simulink model "FINAL_MODEL"  (R2021b)
settings: Solver=VariableStepAuto  StartTime=0.0  StopTime=200  RelTol=1e-3
values from neighbouring files (symbols this model uses):
  lr = 1.6    [projectsetup.m]
  m = 1521    [projectsetup.m]
  posSelector = [1,0,0,0,0,0; 0,0,1,0,0,0]    [projectsetup.m]
  tau = 0.5    [projectsetup.m]
  Ts = 0.1    [projectsetup.m]
  x0_ego = 0    [projectsetup.m]
undefined symbols (not defined in the file or in its folder): AEB, driving
libraries: drivingscenarioandsensors x3, slpidlib x1, trackingutilitieslib x1, drivinglib x1, autolibshared x1
settings Model: Creator=DELL  LastModifiedBy=gioge

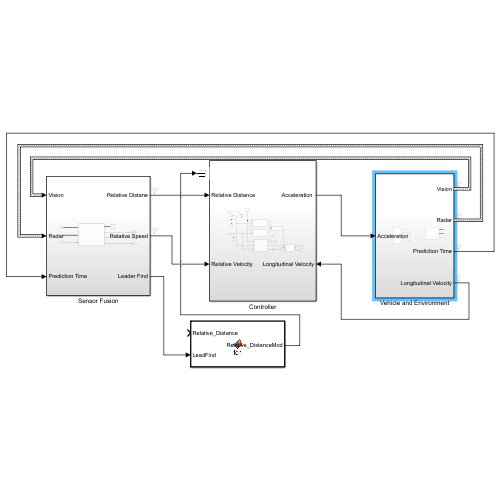
[thumbnail: Simulink's stored preview of the top-level diagram]
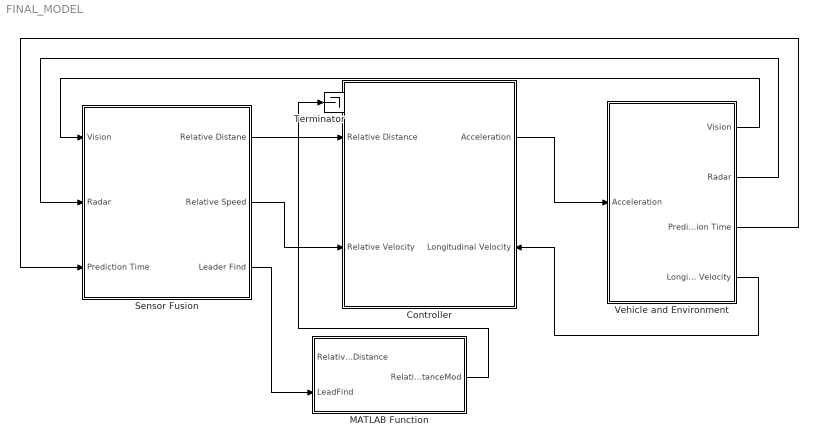
== system FINAL_MODEL ==
  Controller : Subsystem
      settings: PortSchema="{\"entries\":[{\"content\":{\"sides\":[{\"content\":{\"connectorIds\":[\"In1\",\"In2\"]},\"type\":\"ConnectorPlacement.EquallySpacedRectSide\",\"uuid\":\"09646beb-0eff-4bcf-8a55-80fd4dda4f7a\"},{\"content\":{\"connectorIds\":[\"Out1\",\"In3\"],\"side\":\"RIGHT\"},\"type\":\"ConnectorPlacement.EquallySpacedRectSide\",\"uuid\":\"ec392ed6-633f-4d34-b95c-b5fe46f60e49\"},{\"content\":{\"connectorIds\":[],\"side\":\"TOP\"},\"type\":\"ConnectorPlacement.EquallySpacedRectSide\",\"uuid\":\"4c514b4e-b507-45d4-96c7-33bdb79faf54\"},{\"content\":{\"connectorIds\":[],\"side\":\"BOTTOM\"},\"type\":\"ConnectorPlacement.EquallySpacedRectSide\",\"uuid\":\"07bcd855-5437-489d-a027-c45770d5736d\"}]},\"type\":\"ConnectorPlacement.EquallySpacedConnector\",\"uuid\":\"1e09dc8d-e6d5-4259-816a-8e498a37a0b4\"}],\"packageUris\":[\"http://schema.mathworks.com/mf0/Connector/R2020b\"],\"version\":\"1.0\"}"
  MATLAB Function : MATLAB Function  TreatAsAtomicUnit=on
  Sensor Fusion : Subsystem
  Terminator : Terminator
  Vehicle and Environment : Subsystem
  wires:
  Vehicle and Environment/3(Prediction Time) -> Sensor Fusion/3(Prediction Time)
  Vehicle and Environment/2(Radar) -> Sensor Fusion/2(Radar)
  Vehicle and Environment/1(Vision) -> Sensor Fusion/1(Vision)
  Vehicle and Environment/4(Longitudinal Velocity) -> Controller/3(Longitudinal Velocity)
  Sensor Fusion/1(Relative Distane) -> Controller/1(Relative Distance)
  Sensor Fusion/2(Relative Speed) -> Controller/2(Relative Velocity)
  Controller/1("Acceleration ") -> Vehicle and Environment/1(Acceleration)
  Sensor Fusion/3(Leader Find) -> MATLAB Function/2(LeadFind)
  MATLAB Function/1(Relative_DistanceMod) -> Terminator/1

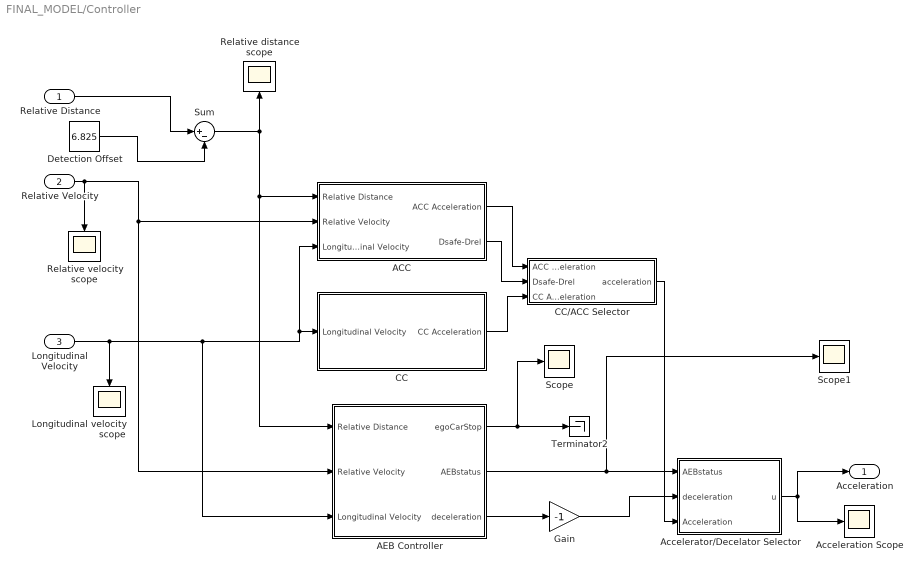
== system FINAL_MODEL/Controller ==
  Relative Distance : Inport
  Relative Velocity : Inport  Port=2
  Longitudinal Velocity : Inport  Port=3
  ACC : Subsystem
  AEB Controller : Subsystem
  Acceleration Scope : Scope
  Accelerator/Decelator Selector : Subsystem
  CC : Subsystem
  CC/ACC Selector : Subsystem
  Detection Offset : Constant  Value=6.825
  Gain : Gain  Gain=-1
  Longitudinal velocity scope : Scope
  Relative distance scope : Scope
  Relative velocity scope : Scope
  Scope : Scope
  Scope1 : Scope
  Sum : Sum  Inputs=|+-
  Terminator2 : Terminator
  "Acceleration " : Outport  OutDataTypeStr=double  PortDimensions=1  SampleTime=[0.10000000000000001,0]  VectorParamsAs1DForOutWhenUnconnected=off
  wires:
  Relative Velocity/1 -> Relative velocity scope/1, AEB Controller/2(Relative Velocity), ACC/2(Relative Velocity)
  Relative Distance/1 -> Sum/1
  AEB Controller/1(egoCarStop) -> Scope/1, Terminator2/1
  AEB Controller/2(AEBstatus) -> Scope1/1, Accelerator/Decelator Selector/1(AEBstatus)
  AEB Controller/3(deceleration) -> Gain/1
  Longitudinal Velocity/1 -> AEB Controller/3(Longitudinal Velocity), ACC/3(Longitudinal Velocity), CC/1(Longitudinal Velocity), Longitudinal velocity scope/1
  Sum/1 -> AEB Controller/1(Relative Distance), ACC/1(Relative Distance), Relative distance scope/1
  Detection Offset/1 -> Sum/2
  Accelerator/Decelator Selector/1(u) -> "Acceleration "/1, Acceleration Scope/1
  Gain/1 -> Accelerator/Decelator Selector/2(deceleration)
  ACC/1(ACC Acceleration) -> CC/ACC Selector/1(ACC Acceleration)
  ACC/2(Dsafe-Drel) -> CC/ACC Selector/2(Dsafe-Drel)
  CC/1(CC Acceleration) -> CC/ACC Selector/3(CC Acceleration)
  CC/ACC Selector/1(acceleration) -> Accelerator/Decelator Selector/3(Acceleration)

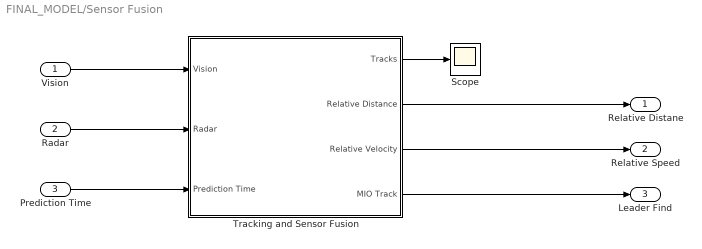
== system FINAL_MODEL/Sensor Fusion ==
  Vision : Inport  OutDataTypeStr=Bus: BusVision  PortDimensions=[1 1]  SampleTime=[0.10000000000000001,0]  BusOutputAsStruct=on
  Radar : Inport  Port=2  OutDataTypeStr=Bus: BusRadar  PortDimensions=[1 1]  SampleTime=[0.10000000000000001,0]  BusOutputAsStruct=on
  Prediction Time : Inport  Port=3  OutDataTypeStr=double  PortDimensions=[1 1]  SampleTime=[0.10000000000000001,0]  BusOutputAsStruct=on
  Scope : Scope
  Tracking and Sensor Fusion : Subsystem  TreatAsAtomicUnit=on
      settings: RTWFileNameOpts=Use function name
  Relative Distane : Outport  OutDataTypeStr=double  PortDimensions=1  SampleTime=[0.10000000000000001,0]  VectorParamsAs1DForOutWhenUnconnected=off  BusOutputAsStruct=on
  Relative Speed : Outport  Port=2  OutDataTypeStr=double  PortDimensions=1  SampleTime=[0.10000000000000001,0]  VectorParamsAs1DForOutWhenUnconnected=off  BusOutputAsStruct=on
  Leader Find : Outport  Port=3  OutDataTypeStr=double  PortDimensions=1  SampleTime=[0.10000000000000001,0]  VectorParamsAs1DForOutWhenUnconnected=off  BusOutputAsStruct=on
  wires:
  Tracking and Sensor Fusion/2(Relative Distance) -> Relative Distane/1
  Prediction Time/1 -> Tracking and Sensor Fusion/3(Prediction Time)
  Tracking and Sensor Fusion/3(Relative Velocity) -> Relative Speed/1
  Tracking and Sensor Fusion/1(Tracks) -> Scope/1
  Radar/1 -> Tracking and Sensor Fusion/2(Radar)
  Vision/1 -> Tracking and Sensor Fusion/1(Vision)
  Tracking and Sensor Fusion/4(MIO Track) -> Leader Find/1

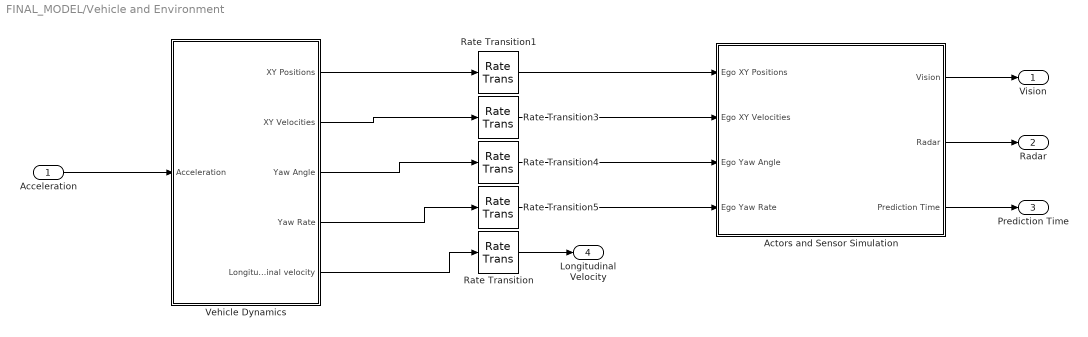
== system FINAL_MODEL/Vehicle and Environment ==
  Acceleration : Inport
  Actors and Sensor Simulation : Subsystem
  Rate Transition{,1,3..5} (5 alike) : RateTransition  OutPortSampleTime=Ts
  Vehicle Dynamics : Subsystem  VariantControl=Variant2
  Vision : Outport  VectorParamsAs1DForOutWhenUnconnected=off
  Radar : Outport  Port=2  VectorParamsAs1DForOutWhenUnconnected=off
  Prediction Time : Outport  Port=3  VectorParamsAs1DForOutWhenUnconnected=off
  Longitudinal Velocity : Outport  Port=4  VectorParamsAs1DForOutWhenUnconnected=off
  wires:
  Acceleration/1 -> Vehicle Dynamics/1(Acceleration)
  Vehicle Dynamics/5(Longitudinal velocity) -> Rate Transition/1
  Vehicle Dynamics/1(XY Positions) -> Rate Transition1/1
  Vehicle Dynamics/3(Yaw Angle) -> Rate Transition4/1
  Actors and Sensor Simulation/1(Vision) -> Vision/1
  Rate Transition/1 -> Longitudinal Velocity/1
  Vehicle Dynamics/2(XY Velocities) -> Rate Transition3/1
  Rate Transition4/1 -> Actors and Sensor Simulation/3(Ego Yaw Angle)
  Actors and Sensor Simulation/2(Radar) -> Radar/1
  Rate Transition1/1 -> Actors and Sensor Simulation/1(Ego XY Positions)
  Rate Transition5/1 -> Actors and Sensor Simulation/4(Ego Yaw Rate)
  Rate Transition3/1 -> Actors and Sensor Simulation/2(Ego XY Velocities)
  Actors and Sensor Simulation/3(Prediction Time) -> Prediction Time/1
  Vehicle Dynamics/4(Yaw Rate) -> Rate Transition5/1

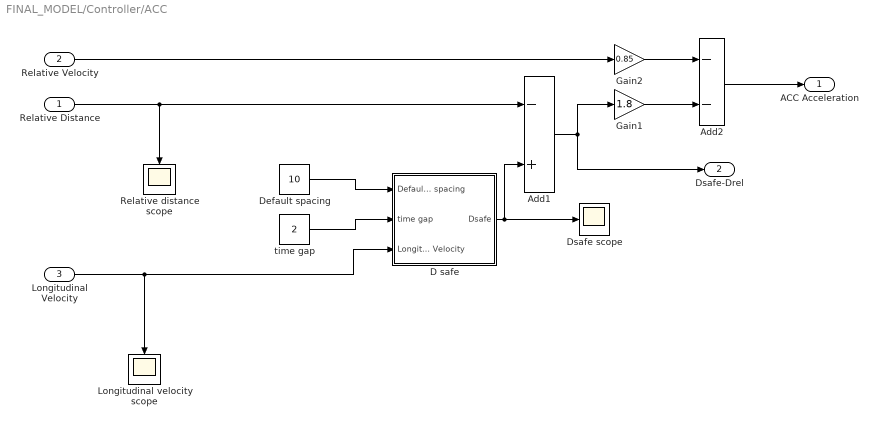
== system FINAL_MODEL/Controller/ACC ==
  Relative Distance : Inport
  Relative Velocity : Inport  Port=2
  Longitudinal Velocity : Inport  Port=3
  Add1 : Sum  Inputs=-+
  Add2 : Sum  Inputs=--
  D safe : Subsystem
  Default spacing : Constant  Value=10
  Dsafe scope : Scope
  Gain1 : Gain  Gain=1.8
  Gain2 : Gain  Gain=0.85
  Longitudinal velocity scope : Scope
  Relative distance scope : Scope
  time gap : Constant  Value=2
  ACC Acceleration : Outport
  Dsafe-Drel : Outport  Port=2
  wires:
  Add1/1 -> Dsafe-Drel/1, Gain1/1
  Relative Distance/1 -> Add1/1, Relative distance scope/1
  D safe/1(Dsafe) -> Add1/2, Dsafe scope/1
  Relative Velocity/1 -> Gain2/1
  time gap/1 -> D safe/2(time gap)
  Longitudinal Velocity/1 -> Longitudinal velocity scope/1, D safe/3(Longitudinal Velocity)
  Default spacing/1 -> D safe/1(Default spacing)
  Gain2/1 -> Add2/1
  Gain1/1 -> Add2/2
  Add2/1 -> ACC Acceleration/1

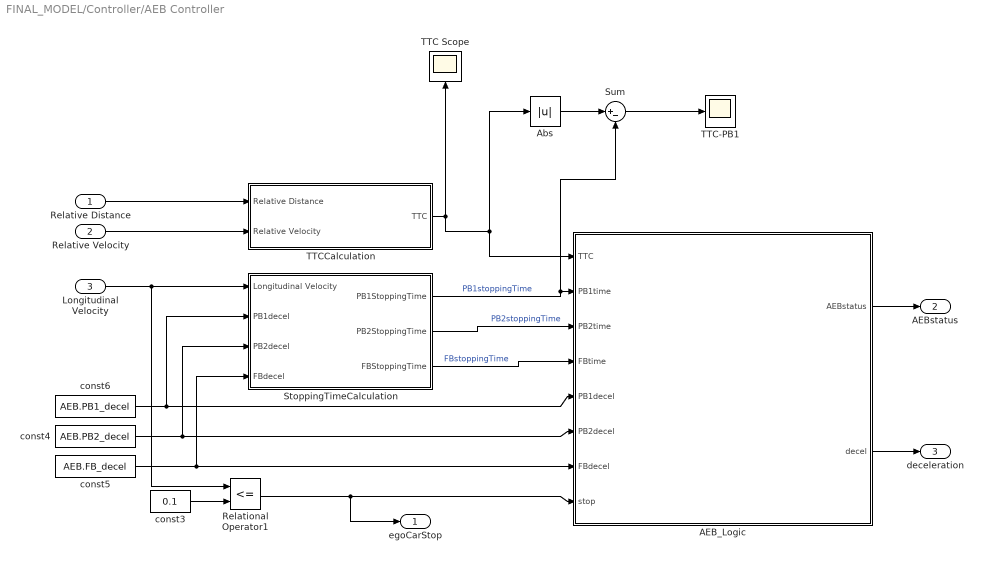
== system FINAL_MODEL/Controller/AEB Controller ==
  Relative Distance : Inport
  Relative Velocity : Inport  Port=2
  Longitudinal Velocity : Inport  Port=3
  AEB_Logic : Stateflow chart  TreatAsAtomicUnit=on
  Abs : Abs
  Relational Operator1 : RelationalOperator  Operator=<=  OutDataTypeStr=boolean  RndMeth=Simplest
  StoppingTimeCalculation : Subsystem
  Sum : Sum  Inputs=|+-
  TTC Scope : Scope
  TTC-PB1 : Scope
  TTCCalculation : Subsystem
  const3 : Constant  Value=0.1  SampleTime=-1
  const4 : Constant  Value=AEB.PB2_decel  SampleTime=-1
  const5 : Constant  Value=AEB.FB_decel  SampleTime=-1
  const6 : Constant  Value=AEB.PB1_decel  SampleTime=-1
  egoCarStop : Outport  VectorParamsAs1DForOutWhenUnconnected=off
  AEBstatus : Outport  Port=2  VectorParamsAs1DForOutWhenUnconnected=off
  deceleration : Outport  Port=3  VectorParamsAs1DForOutWhenUnconnected=off
  wires:
  AEB_Logic/2(decel) -> deceleration/1
  Longitudinal Velocity/1 -> StoppingTimeCalculation/1(Longitudinal Velocity), Relational Operator1/1
  const4/1 -> StoppingTimeCalculation/3(PB2decel), AEB_Logic/6(PB2decel)
  const5/1 -> StoppingTimeCalculation/4(FBdecel), AEB_Logic/7(FBdecel)
  AEB_Logic/1(AEBstatus) -> AEBstatus/1
  const3/1 -> Relational Operator1/2
  Relational Operator1/1 -> egoCarStop/1, AEB_Logic/8(stop)
  const6/1 -> AEB_Logic/5(PB1decel), StoppingTimeCalculation/2(PB1decel)
  StoppingTimeCalculation/2(PB2StoppingTime) -> AEB_Logic/3(PB2time)  "PB2stoppingTime"
  StoppingTimeCalculation/1(PB1StoppingTime) -> Sum/2, AEB_Logic/2(PB1time)  "PB1stoppingTime"
  StoppingTimeCalculation/3(FBStoppingTime) -> AEB_Logic/4(FBtime)  "FBstoppingTime"
  Relative Distance/1 -> TTCCalculation/1(Relative Distance)
  Relative Velocity/1 -> TTCCalculation/2(Relative Velocity)
  TTCCalculation/1(TTC) -> Abs/1, AEB_Logic/1(TTC), TTC Scope/1
  Abs/1 -> Sum/1
  Sum/1 -> TTC-PB1/1

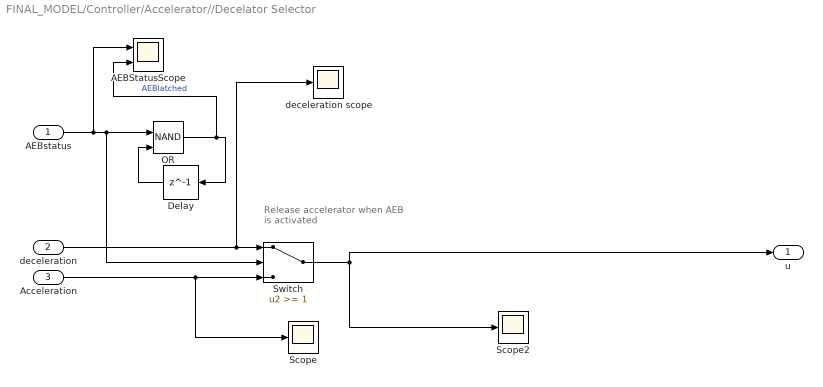
== system FINAL_MODEL/Controller/Accelerator//Decelator Selector ==
  note: Release accelerator when AEB is activated
  AEBstatus : Inport
  deceleration : Inport  Port=2
  Acceleration : Inport  Port=3
  AEBStatusScope : Scope  NumInputPorts=2
  Delay : Delay  DelayLength=1
  OR : Logic  Operator=NAND  IconShape=distinctive  AllPortsSameDT=off  OutDataTypeStr=boolean
  Scope : Scope
  Scope2 : Scope
  Switch : Switch  Threshold=1
  deceleration scope : Scope
  u : Outport  VectorParamsAs1DForOutWhenUnconnected=off
  wires:
  OR/1 -> AEBStatusScope/2, Delay/1  "AEBlatched"
  Delay/1 -> OR/2
  Switch/1 -> Scope2/1, u/1
  AEBstatus/1 -> AEBStatusScope/1, Switch/2, OR/1
  deceleration/1 -> deceleration scope/1, Switch/1
  Acceleration/1 -> Scope/1, Switch/3

== system FINAL_MODEL/Controller/CC ==
  Longitudinal Velocity : Inport
  Add : Sum  Inputs=-+
  Longitudinal velocity scope : Scope
  PID Controller : slpidlib/PID Controller  Controller=P  Form=Parallel  TimeDomain=Continuous-time  UseExternalTs=off  SampleTime=-1  IntegratorMethod=Forward Euler  FilterMethod=Forward Euler  ControllerParametersSource=internal  P=0.5  I=0.01  D=0  UseFilter=on  N=100  TunerSelectOption=Transfer Function Based (PID Tuner App)  InitialConditionSource=internal  InitialConditionForIntegrator=0  InitialConditionForFilter=0  DifferentiatorICPrevScaledInput=0  ExternalReset=none  TrackingMode=off  Kt=1  LimitOutput=off  SatLimitsSource=internal  UpperSaturationLimit=2  LowerSaturationLimit=-3  LinearizeAsGain=on  AntiWindupMode=none  Kb=1  POutMin=[]  POutMax=[]  IOutMin=[]  IOutMax=[]  DOutMin=[]  DOutMax=[]  NOutMin=[]  NOutMax=[]  SumOutMin=[]  SumOutMax=[]  SaturationOutMin=[]  SaturationOutMax=[]  PParamMin=[]  PParamMax=[]  IParamMin=[]  IParamMax=[]  DParamMin=[]  DParamMax=[]  NParamMin=[]  NParamMax=[]  KbParamMin=[]  KbParamMax=[]  KtParamMin=[]  KtParamMax=[]  KbOutMin=[]  KbOutMax=[]  KtOutMin=[]  KtOutMax=[]  IntegratorOutMin=[]  IntegratorOutMax=[]  FilterOutMin=[]  FilterOutMax=[]  SumI1OutMin=[]  SumI1OutMax=[]  SumI2OutMin=[]  SumI2OutMax=[]  SumI3OutMin=[]  SumI3OutMax=[]  SumI4OutMin=[]  SumI4OutMax=[]  SumDOutMin=[]  SumDOutMax=[]  DifferentiatorOutMin=[]  DifferentiatorOutMax=[]  FilterDiffOutCoefMin=[]  FilterDiffOutCoefMax=[]  ReciprocalOutMin=[]  ReciprocalOutMax=[]  SumDenOutMin=[]  SumDenOutMax=[]  SumNumOutMin=[]  SumNumOutMax=[]  DivideOutMin=[]  DivideOutMax=[]  UdiffTsProdOutMin=[]  UdiffTsProdOutMax=[]  NTsProdOutMin=[]  NTsProdOutMax=[]  UintegralTsProdOutMin=[]  UintegralTsProdOutMax=[]  UngainTsProdOutMin=[]  UngainTsProdOutMax=[]  IntegratorContinuousStateAttributes=''  IntegratorStateMustResolveToSignalObject=off  IntegratorRTWStateStorageClass=Auto  FilterContinuousStateAttributes=''  FilterStateMustResolveToSignalObject=off  FilterRTWStateStorageClass=Auto  ParallelPVariant=InternalParameters  IdealPVariant=Disabled  IVariant=Disabled  DVariant=Disabled  IntegratorVariant=Disabled  SatVariant=Disabled  AWVariant=Disabled  PCopyVariant=Disabled  TRVariant=Disabled  FdbkBlocksVariant=Forward  IdealPFdbkVariant=Disabled  SatFdbkVariant=Disabled  DerivativeFilterVariant=Disabled  NVariant=Disabled  NCopyVariant=Disabled_SignalSpec  FilterICVariant=Disabled  IntegratorICVariant=Disabled  ExternalResetVariant=Disabled  TRSumVariant=Passthrough  SumFdbkVariant=Disabled  SumVariant=Passthrough_P  TsampFilterVariant=InternalTs  TsampNgainVariant=Passthrough  TsampIntegralVariant=Disabled_SignalSpec  ExternalSaturationOutDataTypeStr=Inherit: Same as second input
  PID scope : Scope
  set velocity : Constant  Value=18
  CC Acceleration : Outport
  wires:
  PID Controller/1 -> CC Acceleration/1, PID scope/1
  set velocity/1 -> Add/2
  Longitudinal Velocity/1 -> Longitudinal velocity scope/1, Add/1
  Add/1 -> PID Controller/1

== system FINAL_MODEL/Controller/CC//ACC Selector ==
  ACC Acceleration : Inport
  Dsafe-Drel : Inport  Port=2
  CC Acceleration : Inport  Port=3
  Min1 : MinMax  Inputs=2
  Saturation : Saturate  UpperLimit=2  LowerLimit=-5
  Switch : Switch  Criteria=u2 > Threshold
  acceleration : Outport
  wires:
  ACC Acceleration/1 -> Min1/1, Switch/1
  Saturation/1 -> acceleration/1
  Switch/1 -> Saturation/1
  CC Acceleration/1 -> Min1/2
  Dsafe-Drel/1 -> Switch/2
  Min1/1 -> Switch/3

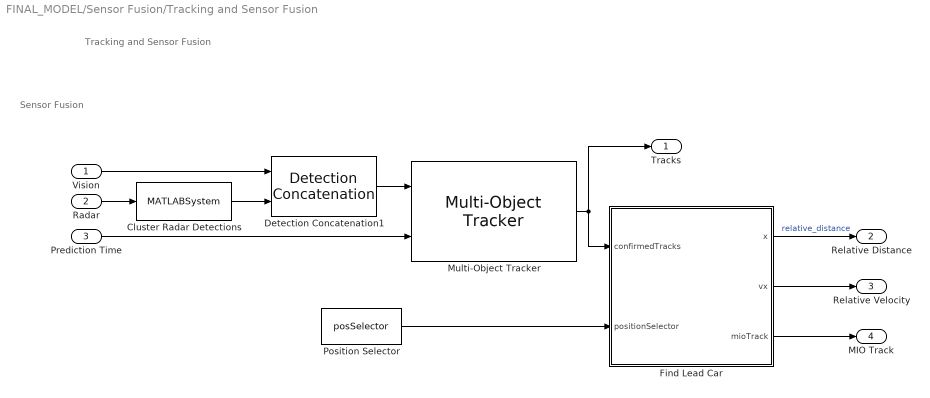
== system FINAL_MODEL/Sensor Fusion/Tracking and Sensor Fusion ==
  note: Sensor Fusion
  note: Tracking and Sensor Fusion
  Vision : Inport  OutDataTypeStr=Bus: BusVision  PortDimensions=[1 1]  SampleTime=[0.10000000000000001,0]  BusOutputAsStruct=on
  Radar : Inport  Port=2  OutDataTypeStr=Bus: BusRadar  PortDimensions=[1 1]  SampleTime=[0.10000000000000001,0]  BusOutputAsStruct=on
  Prediction Time : Inport  Port=3  OutDataTypeStr=double  PortDimensions=[1 1]  SampleTime=[0.10000000000000001,0]  BusOutputAsStruct=on
  Cluster Radar Detections : MATLABSystem  System=helperClusterDetections  ClusterSize=clusterSize  BusNameSource=Auto  BusName=BusClusterDetections  SimulateUsing=Interpreted execution
      mask Type: helperClusterDetections
      mask Display:
      | disp(['Detection' char(10) 'Clustering']);
      | port_label('input',1,'In');
      | port_label('output',1,'Out');
  Detection Concatenation1 : trackingutilitieslib/Detection Concatenation  NumInputs=2  BusNameSource=Auto  BusName=BusDetectionConcatenation1  SimulateUsing=Interpreted execution
      settings: SourceProductBaseCode=AE,DR,TF,RA,UV,VE
  Find Lead Car : MATLAB Function  TreatAsAtomicUnit=on
  Multi-Object Tracker : drivinglib/Multi-Object Tracker  TrackerIndex=uint32( 0 )  FilterInitializationFcn=initcvekf  AssignmentThreshold=assigThresh  ConfirmationThreshold=[ 2, 3 ]  DeletionThreshold=[ 5, 5 ]  MaxNumTracks=numTracks  MaxNumSensors=numSensors  OOSMHandling=Terminate  StateParametersSimulink=struct  HasStateParametersInput=off  TimeInputSource=Input port  HasCostMatrixInput=off  HasDetectableTrackIDsInput=off  BusNameSource=Property  BusName=BusMultiObjectTracker1  TentativeTracksOutputPort=off  AllTracksOutputPort=off  SimulateUsing=Interpreted execution
      settings: SourceProductBaseCode=DR
  Position Selector : Constant  Value=posSelector
  Tracks : Outport  OutDataTypeStr=Bus:BusMultiObjectTracker1  PortDimensions=[1 1]  SampleTime=[0.10000000000000001,0]  VectorParamsAs1DForOutWhenUnconnected=off  BusOutputAsStruct=on
  Relative Distance : Outport  Port=2  VectorParamsAs1DForOutWhenUnconnected=off
  Relative Velocity : Outport  Port=3  VectorParamsAs1DForOutWhenUnconnected=off
  MIO Track : Outport  Port=4  VectorParamsAs1DForOutWhenUnconnected=off
  wires:
  Find Lead Car/3(mioTrack) -> MIO Track/1
  Cluster Radar Detections/1 -> Detection Concatenation1/2
  Vision/1 -> Detection Concatenation1/1
  Prediction Time/1 -> Multi-Object Tracker/2
  Find Lead Car/2(vx) -> Relative Velocity/1
  Radar/1 -> Cluster Radar Detections/1
  Multi-Object Tracker/1 -> Find Lead Car/1(confirmedTracks), Tracks/1
  Detection Concatenation1/1 -> Multi-Object Tracker/1
  Find Lead Car/1(x) -> Relative Distance/1  "relative_distance"
  Position Selector/1 -> Find Lead Car/2(positionSelector)

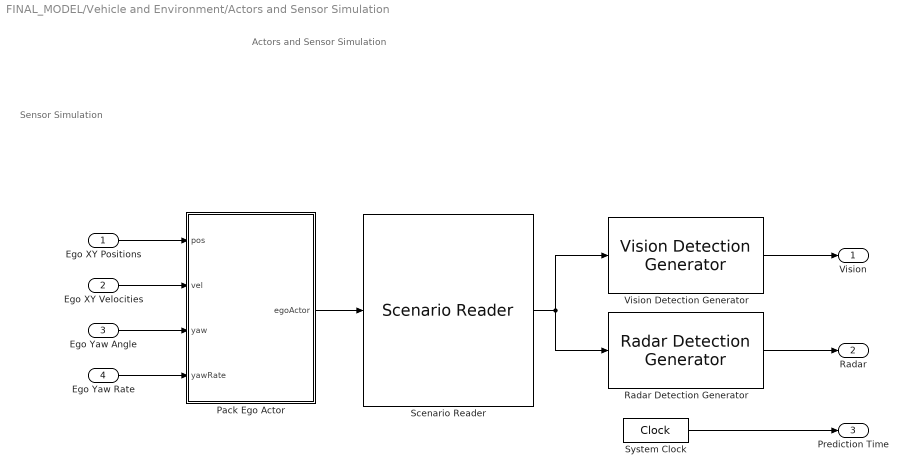
== system FINAL_MODEL/Vehicle and Environment/Actors and Sensor Simulation ==
  note: Sensor Simulation
  note: Actors and Sensor Simulation
  Ego XY Positions : Inport
  Ego XY Velocities : Inport  Port=2
  Ego Yaw Angle : Inport  Port=3
  Ego Yaw Rate : Inport  Port=4
  Pack Ego Actor : MATLAB Function  TreatAsAtomicUnit=on
  Radar Detection Generator : drivingscenarioandsensors/Radar Detection Generator  SensorIndex=2  UpdateInterval=0.1  SensorLocation=[ 3.7, 0 ]  Height=0.2  Yaw=0  Pitch=0  Roll=0  BusNameSource=Property  BusName=BusRadar  MaxNumDetectionsSource=Property  MaxNumDetections=50  DetectionCoordinates=Ego Cartesian  SimulateUsing=Interpreted execution  AzimuthResolution=4  ElevationResolution=10  RangeResolution=2.5  RangeRateResolution=0.5  AzimuthBiasFraction=0.1  ElevationBiasFraction=0.1  RangeBiasFraction=0.05  RangeRateBiasFraction=0.05  FieldOfView=[ 20, 5 ]  MaxRange=174  RangeRateLimits=[ -100, 100 ]  DetectionProbability=0.9  FalseAlarmRate=1e-6  ReferenceRange=100  ReferenceRCS=0  HasElevation=off  HasRangeRate=on  HasNoise=off  HasFalseAlarms=off  HasOcclusion=on  InitialSeedSource=Repeatable  InitialSeed=0  UsedSeed=driving.internal.SimulinkUtilities.seedManager(gcb)  ActorProfilesSource=Parameters  ActorProfilesParameters=driving.internal.ActorProfilesRadarParameters  ActorProfilesExpression=struct( 'ClassID', 0, 'Length', 4.7, 'Width', 1.8, 'Height', 1.4, 'OriginOffset', [ -1.35, 0, 0 ], 'RCSPattern', [ 10, 10; 10, 10 ], 'RCSAzimuthAngles', [ -180, 180 ], 'RCSElevationAngles', [ -90, 90 ] )
      settings: SourceProductBaseCode=DR
  Scenario Reader : drivingscenarioandsensors/Scenario Reader  ScenarioSource=From file  ScenarioFileName=C:\Users\gioge\OneDrive\Desktop\Tesi\MODELLO\Prova.mat  ScenarioVariableName=scenario  OutputCoordinateSystem=Vehicle coordinates  EgoVehicleSource=Input port  EgoVehicleActorID=1  OrientVehiclesOnRoad=off  OutputEgoVehiclePose=off  OutputEgoVehicleState=off  SampleTime=0.1  LaneBoundaryOutput=None  LaneBoundaryDistance=0:0.5:9.5  LaneBoundaryLocation=Center of lane markings  BusNameSource=Property  BusName=BusActors  BusNumActorsSource=Scenario  BusNumActors=100  BusName2Source=Auto  BusName2=BusLaneBoundaries  BusNumLaneBoundariesSource=Scenario  BusNumLaneBoundaries=10  BusName3Source=Auto  BusName3=BusEgoActor  BusName4Source=Auto  BusName4=BusEgoState  ShowCoordinateLabels=on  SimulateUsing=Interpreted execution
  System Clock : DigitalClock  SampleTime=Ts
  Vision Detection Generator : drivingscenarioandsensors/Vision Detection Generator  SensorIndex=1  DetectorOutput=Objects only  UpdateInterval=0.1  LaneUpdateInterval=0.1  SensorLocation=[ 2.1, 0 ]  Height=1.1  Yaw=0  Pitch=1  Roll=0  BusNameSource=Property  BusName=BusVision  BusName2Source=Auto  BusName2=BusLaneDetections  MaxNumDetectionsSource=Property  MaxNumDetections=20  MaxNumLanesSource=Property  MaxNumLanes=30  DetectionCoordinates=Ego Cartesian  SimulateUsing=Interpreted execution  MaxRange=150  BoundingBoxAccuracy=5  ProcessNoiseIntensity=5  MaxSpeed=50  MaxAllowedOcclusion=0.5  MinObjectImageSize=[ 15, 15 ]  DetectionProbability=0.9  FalsePositivesPerImage=0.1  MinLaneImageSize=[ 20, 5 ]  LaneBoundaryAccuracy=3  HasNoise=off  InitialSeedSource=Repeatable  InitialSeed=0  UsedSeed=driving.internal.SimulinkUtilities.seedManager(gcb)  ActorProfilesSource=Parameters  ActorProfilesParameters=driving.internal.ActorProfilesParameters  ActorProfilesExpression=struct( 'ClassID', 0, 'Length', 4.7, 'Width', 1.8, 'Height', 1.4, 'OriginOffset', [ -1.35, 0, 0 ] )  Intrinsics=driving.internal.cameraIntrinsics
  Vision : Outport  VectorParamsAs1DForOutWhenUnconnected=off
  Radar : Outport  Port=2  VectorParamsAs1DForOutWhenUnconnected=off
  Prediction Time : Outport  Port=3  VectorParamsAs1DForOutWhenUnconnected=off
  wires:
  Scenario Reader/1 -> Radar Detection Generator/1, Vision Detection Generator/1
  Vision Detection Generator/1 -> Vision/1
  System Clock/1 -> Prediction Time/1
  Pack Ego Actor/1(egoActor) -> Scenario Reader/1
  Radar Detection Generator/1 -> Radar/1
  Ego XY Positions/1 -> Pack Ego Actor/1(pos)
  Ego XY Velocities/1 -> Pack Ego Actor/2(vel)
  Ego Yaw Angle/1 -> Pack Ego Actor/3(yaw)
  Ego Yaw Rate/1 -> Pack Ego Actor/4(yawRate)

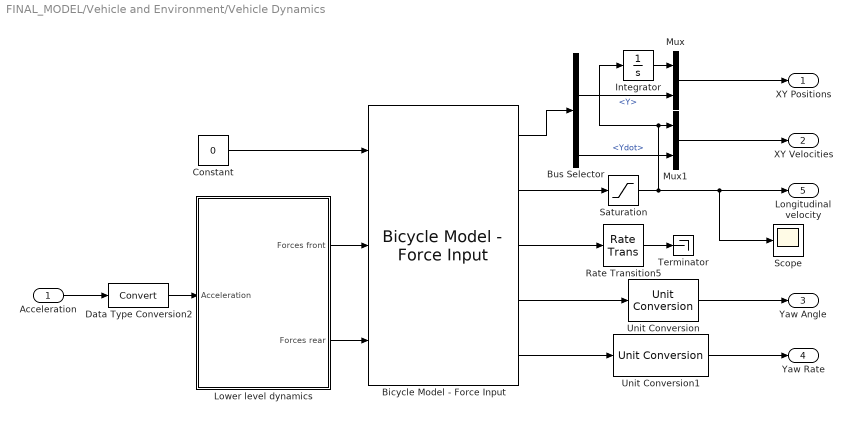
== system FINAL_MODEL/Vehicle and Environment/Vehicle Dynamics ==
  Acceleration : Inport  Unit=m/s^2
  Bicycle Model - Force Input : autolibshared/Bicycle Model - Force Input  trackMode=Single (bicycle)  inputMode=External longitudinal forces  frontSteerMode=on  rearSteerMode=off  windMode=off  muMode=off  extFMode=off  extMMode=off  aMode=3  NF=2  NR=2  m=m  a=lf  b=lr  h=0.35  X_o=x0_ego  xdot_o=v0_ego  CalphaMode=off  sigmaMode=on  w=[1.4,1.4]  Cy_f=Cf  Cy_r=Cr  sigma_f=.1  sigma_r=.1  alpha_f_brk=[-.1 .1]  Cy_f_data=[-9e3 9e3]  alpha_r_brk=[-.1 .1]  Cy_r_data=[-9e3 9e3]  Y_o=y0_ego  ydot_o=0  Izz=Iz  psi_o=0  r_o=0  Af=0  Cd=.3  Cl=.1  Cpm=.1  beta_w=[0:0.01:0.3]  Cs=[0:0.03:0.9]  Cym=[0:0.01:0.3]  Pabs=101325  Tair=273  g=9.81  mu=1  xdot_tol=.01  Fznom=5000  Fxtire_sat=1e6  Fytire_sat=1e6  longOff=0  latOff=0  vertOff=0
      settings: SourceProductBaseCode=PW,DR,MT,UV,VE
  Bus Selector : BusSelector  OutputSignals=InertFrm.FrntAxl.Disp.X,InertFrm.FrntAxl.Disp.Y,InertFrm.FrntAxl.Vel.Xdot,InertFrm.FrntAxl.Vel.Ydot
  Constant : Constant  Value=0  SampleTime=0.1
  Data Type Conversion2 : DataTypeConversion
  Integrator : Integrator  InitialCondition=x0_ego
  Lower level dynamics : Subsystem
  Mux : Mux  Inputs=2
  Mux1 : Mux  Inputs=2
  Rate Transition5 : RateTransition  OutPortSampleTime=Ts
  Saturation : Saturate  UpperLimit=100  LowerLimit=0
  Scope : Scope
  Terminator : Terminator
  Unit Conversion : UnitConversion
  Unit Conversion1 : UnitConversion
  XY Positions : Outport  Unit=m  VectorParamsAs1DForOutWhenUnconnected=off
  XY Velocities : Outport  Port=2  Unit=m/s  VectorParamsAs1DForOutWhenUnconnected=off
  Yaw Angle : Outport  Port=3  Unit=deg  VectorParamsAs1DForOutWhenUnconnected=off
  Yaw Rate : Outport  Port=4  Unit=degree/s  VectorParamsAs1DForOutWhenUnconnected=off
  Longitudinal velocity : Outport  Port=5  VectorParamsAs1DForOutWhenUnconnected=off
  wires:
  Lower level dynamics/2(Forces rear) -> Bicycle Model - Force Input/3
  Lower level dynamics/1(Forces front) -> Bicycle Model - Force Input/2
  Data Type Conversion2/1 -> Lower level dynamics/1(Acceleration)
  Acceleration/1 -> Data Type Conversion2/1
  Bicycle Model - Force Input/4 -> Unit Conversion/1
  Bus Selector/4 -> Mux1/2  "<Ydot>"
  Bus Selector/2 -> Mux/2  "<Y>"
  Bicycle Model - Force Input/1 -> Bus Selector/1
  Mux/1 -> XY Positions/1
  Mux1/1 -> XY Velocities/1
  Bicycle Model - Force Input/5 -> Unit Conversion1/1
  Unit Conversion/1 -> Yaw Angle/1
  Unit Conversion1/1 -> Yaw Rate/1
  Bicycle Model - Force Input/3 -> Rate Transition5/1
  Rate Transition5/1 -> Terminator/1
  Constant/1 -> Bicycle Model - Force Input/1
  Bicycle Model - Force Input/2 -> Saturation/1
  Saturation/1 -> Integrator/1, Mux1/1, Scope/1, Longitudinal velocity/1
  Integrator/1 -> Mux/1

== system FINAL_MODEL/Controller/ACC/D safe ==
  Default spacing : Inport
  time gap : Inport  Port=2
  Longitudinal Velocity : Inport  Port=3
  Add : Sum
  Product : Product
  Scope : Scope
  Dsafe : Outport
  wires:
  Longitudinal Velocity/1 -> Product/1
  time gap/1 -> Product/2
  Product/1 -> Add/2
  Default spacing/1 -> Add/1
  Add/1 -> Scope/1, Dsafe/1

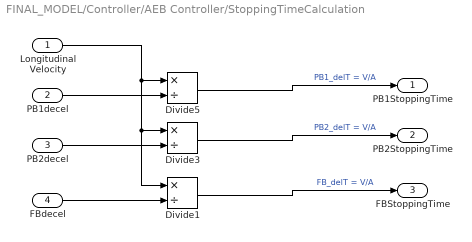
== system FINAL_MODEL/Controller/AEB Controller/StoppingTimeCalculation ==
  Longitudinal Velocity : Inport
  PB1decel : Inport  Port=2
  PB2decel : Inport  Port=3
  FBdecel : Inport  Port=4
  Divide1 : Product  Inputs=*/
  Divide3 : Product  Inputs=*/
  Divide5 : Product  Inputs=*/
  PB1StoppingTime : Outport  VectorParamsAs1DForOutWhenUnconnected=off
  PB2StoppingTime : Outport  Port=2  VectorParamsAs1DForOutWhenUnconnected=off
  FBStoppingTime : Outport  Port=3  VectorParamsAs1DForOutWhenUnconnected=off
  wires:
  Longitudinal Velocity/1 -> Divide1/1, Divide3/1, Divide5/1
  Divide5/1 -> PB1StoppingTime/1  "PB1_delT = V/A"
  Divide1/1 -> FBStoppingTime/1  "FB_delT = V/A"
  PB1decel/1 -> Divide5/2
  PB2decel/1 -> Divide3/2
  FBdecel/1 -> Divide1/2
  Divide3/1 -> PB2StoppingTime/1  "PB2_delT = V/A"

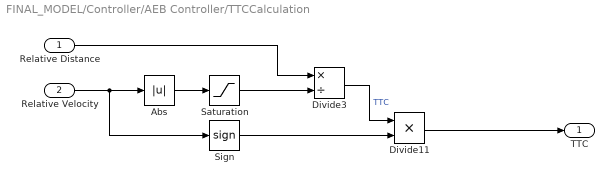
== system FINAL_MODEL/Controller/AEB Controller/TTCCalculation ==
  Relative Distance : Inport
  Relative Velocity : Inport  Port=2
  Abs : Abs
  Divide11 : Product  Inputs=**
  Divide3 : Product  Inputs=*/
  Saturation : Saturate  UpperLimit=100  LowerLimit=0.01
  Sign : Signum
  TTC : Outport  VectorParamsAs1DForOutWhenUnconnected=off
  wires:
  Relative Velocity/1 -> Sign/1, Abs/1
  Divide3/1 -> Divide11/1  "TTC"
  Abs/1 -> Saturation/1
  Saturation/1 -> Divide3/2
  Sign/1 -> Divide11/2
  Divide11/1 -> TTC/1
  Relative Distance/1 -> Divide3/1

== system FINAL_MODEL/Vehicle and Environment/Vehicle Dynamics/Lower level dynamics ==
  Acceleration : Inport
  Gain : Gain  Gain=m
  Gain1 : Gain  Gain=0.5
  Lower level dynamics : TransferFcn  Denominator=[tau 1]
  Forces front : Outport  VectorParamsAs1DForOutWhenUnconnected=off
  Forces rear : Outport  Port=2  VectorParamsAs1DForOutWhenUnconnected=off
  wires:
  Gain/1 -> Gain1/1
  Gain1/1 -> Forces front/1, Forces rear/1
  Acceleration/1 -> Lower level dynamics/1
  Lower level dynamics/1 -> Gain/1

== matlab function FINAL_MODEL/MATLAB Function ==
  data: Relative_Distance input; LeadFind input; Relative_DistanceMod output
function Relative_DistanceMod = fcn(Relative_Distance, LeadFind)
if LeadFind == 0
    Relative_DistanceMod = 70;
else
    Relative_DistanceMod = Relative_Distance;

end

== matlab function FINAL_MODEL/Vehicle and Environment/Actors and Sensor Simulation/Pack Ego Actor ==
  data: pos input; egoActor output Bus: BusActorsActors size=1; vel input; yaw input; yawRate input
function egoActor = packEgo(pos,vel,yaw,yawRate)
% Pack ego information into a single ego actor bus
%
% Imoprtant note:
% Output is a bus of type BusActorsActors. This is the same bus used by the
% Scenario Reader to output an individual actor. If you change the
% output bus name of Scenario Reader, change the output bus name here
% as well by clicking on 'Edit Data' in the menu above.

egoActor = struct(...
    'ActorID',1,...
    'Position', [pos(1) pos(2) 0], ...
    'Velocity', [vel(1) vel(2) 0], ...
    'Roll', 0, ...
    'Pitch', 0, ...
    'Yaw', yaw, ...
    'AngularVelocity', [0 0 yawRate]);

== matlab function FINAL_MODEL/Sensor Fusion/Tracking and Sensor Fusion/Find Lead Car ==
  data: confirmedTracks input; x output double size=[1 1]; vx output size=[1 1]; mioTrack output; positionSelector input
function [x,vx,mioTrack] = findLeadCar(confirmedTracks, positionSelector)
% This function finds the lead car: a car in front of the ego car that
% satisfies all the criteria below:
% * Within the ego car's lane.
% * In front of the ego car.
% * Closest to the ego car.

% Important notes:
% 1. If you change state definition, change the following:
%       State = [x;vx;y;vy;z;vz] (3D constant velocity)
curvature = 1/1000000000000000000;
numStates = 6;

% 2. The lane is defined using a parabolic model, where y=ax^2+bx+c. a is
%    equal to half the road curvature, b=0, and c is the offset of the lane
%    boundaries relative to the ego car. Overall lane width is assumed to
%    be 3.6m, typical highway lane width.
laneWidth = 3.6;

% 3. The ego car is assumed to be traveling in the middle of its lane, with
%    1.8m on each side of it. So, c=+1.8m for the left lane boundary and
%    -1.8m for the right lane boundary.
halfLaneWidth = laneWidth/2;

% Initialize outputs and parameters
maxX = cast(1000, 'like', confirmedTracks.Tracks(1).State);  % Far enough forward so that no track is expected to exceed this distance
trackID = 0;

for i = 1:confirmedTracks.NumTracks
    position = positionSelector * confirmedTracks.Tracks(i).State;
    x = position(1); % Longitudinal position of the track relative to ego
    y = position(2); % Lateral position of the track relative to ego
    
    if x < maxX && x > 0 % No point checking otherwise
        yleftLane  = polyval([curvature/2, 0,  halfLaneWidth],x); % Half a lane to the left
        yrightLane = polyval([curvature/2, 0, -halfLaneWidth],x); % Half a lane to the right
        
        % Find a new lead car
        if (yrightLane <= y) && (y <= yleftLane)
            maxX = x;
            trackID = i;
        end
    end
end

if trackID>0
    mioState = confirmedTracks.Tracks(trackID).State;
else
    mioState = inf(numStates,1,'like',confirmedTracks.Tracks(1).State);
end

% Output:
x = mioState(1);    % Longitudinal position of the lead car
vx = mioState(2);   % Longitudinal velocity of the lead car
mioTrack = trackID; % Index of the most important track

== stateflow chart FINAL_MODEL/Controller/AEB Controller/AEB_Logic ==
  note: AEB Logic
  state Default
    entry: AEBstatus = 0;
    decel = 0;
  state Partial_Braking1
    entry: AEBstatus = 1;
    decel = PB1decel;
  state Full_Braking
    entry: AEBstatus = 3;
    decel = FBdecel;
  state Partial_Braking2
    entry: AEBstatus = 2;
    decel = PB2decel;
  (default) -> Default
  Full_Braking -> Default : [stop==1]
  Partial_Braking1 -> Default [order 2] : [stop==1]
  Partial_Braking2 -> Default [order 2] : [stop==1]
  Default -> Partial_Braking1 : [(abs(TTC) < PB1time) && TTC<0]
  Partial_Braking1 -> Partial_Braking2 [order 1] : [(abs(TTC) < PB2time) && TTC<0]
  Partial_Braking2 -> Full_Braking [order 1] : [(abs(TTC) < FBtime) && TTC<0]
  data: TTC input; PB1time input; PB2time input; FBtime input; PB1decel input; PB2decel input; FBdecel input; AEBstatus output; decel output; stop input
